simulink library "csu_lnh_ln200_hardware_lib_a"  (R2014b)
settings: Solver=ode45  SolverMode=SingleTasking  StartTime=0.0  StopTime=10.0  RelTol=1e-3
undefined symbols (not defined in the file or in its folder): lnh_accel_range, lnh_accel_SF, lnh_correlation_time, lnh_dt, lnh_gyro_g_sensitive, lnh_gyro_range, lnh_gyro_SF, lnh_gyro_vibe_sensitive
libraries: util_common_lib x7, util_tf_lib x2, util_info_lib x1
settings Model: Creator=hcannon  LastModifiedBy=mstewart

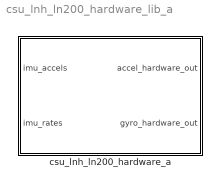
== system csu_lnh_ln200_hardware_lib_a ==
  csu_lnh_ln200_hardware_a : Subsystem

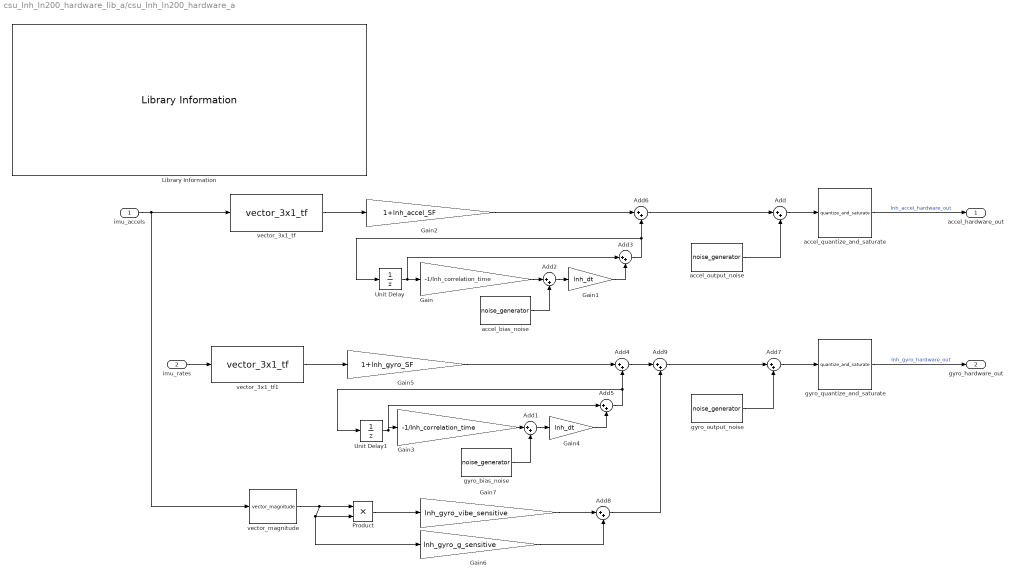
== system csu_lnh_ln200_hardware_lib_a/csu_lnh_ln200_hardware_a ==
  imu_accels : Inport
  imu_rates : Inport  Port=2
  Add{,1..9} (10 alike) : Sum  Inputs=|++
  Gain : Gain  Gain=-1/lnh_correlation_time
  Gain1 : Gain  Gain=lnh_dt
  Gain2 : Gain  Gain=1+lnh_accel_SF
  Gain3 : Gain  Gain=-1/lnh_correlation_time
  Gain4 : Gain  Gain=lnh_dt
  Gain5 : Gain  Gain=1+lnh_gyro_SF
  Gain6 : Gain  Gain=lnh_gyro_g_sensitive
  Gain7 : Gain  Gain=lnh_gyro_vibe_sensitive
  Library Information : util_info_lib/Library Information  owner='NONE'
  Product : Product  RndMeth=Zero
  Unit Delay : UnitDelay  SampleTime=-1
  Unit Delay1 : UnitDelay  SampleTime=-1
  accel_bias_noise : util_common_lib/noise_generator  std_dev=lnh_accel_bias_noise_v  bias=lnh_accel_bias_bias_v  seed=lnh_accel_bias_seed_v  on=lnh_accel_noise_on  sample_time=sim_time_step_size
  accel_output_noise : util_common_lib/noise_generator  std_dev=lnh_accel_noise_v  bias=lnh_accel_bias_v  seed=lnh_accel_seed_v  on=lnh_accel_noise_on  sample_time=sim_time_step_size
  accel_quantize_and_saturate : util_common_lib/quantize_and_saturate  RES=lnh_accel_sensitivity  OPER=truncate  out_min=-lnh_accel_range  out_max=lnh_accel_range
  gyro_bias_noise : util_common_lib/noise_generator  std_dev=lnh_gyro_bias_noise_v  bias=lnh_gyro_bias_bias_v  seed=lnh_gyro_bias_seed_v  on=lnh_gyro_noise_on  sample_time=sim_time_step_size
  gyro_output_noise : util_common_lib/noise_generator  std_dev=lnh_gyro_noise_v  bias=lnh_gyro_bias_v  seed=lnh_gyro_seed_v  on=lnh_gyro_noise_on  sample_time=sim_time_step_size
  gyro_quantize_and_saturate : util_common_lib/quantize_and_saturate  RES=lnh_gyro_sensitivity  OPER=truncate  out_min=-lnh_gyro_range  out_max=lnh_gyro_range
  vector_3x1_tf : util_tf_lib/vector_3x1_tf  num=lnh_accel_response_num  den=lnh_accel_response_den  st=-1
  vector_3x1_tf1 : util_tf_lib/vector_3x1_tf  num=lnh_gyro_response_num  den=lnh_gyro_response_den  st=-1
  vector_magnitude : util_common_lib/vector_magnitude  SystemSampleTime=-1
  accel_hardware_out : Outport
  gyro_hardware_out : Outport  Port=2
  wires:
  Add8/1 -> Add9/2
  Add9/1 -> Add7/1
  Add4/1 -> Add9/1
  Gain6/1 -> Add8/2
  Gain7/1 -> Add8/1
  Product/1 -> Gain7/1
  vector_magnitude/1 -> Gain6/1, Product/2, Product/1
  Add6/1 -> Add/1
  Gain2/1 -> Add6/1
  Gain5/1 -> Add4/1
  Add/1 -> accel_quantize_and_saturate/1
  accel_quantize_and_saturate/1 -> accel_hardware_out/1  "lnh_accel_hardware_out"
  gyro_quantize_and_saturate/1 -> gyro_hardware_out/1  "lnh_gyro_hardware_out"
  imu_accels/1 -> vector_magnitude/1, vector_3x1_tf/1
  imu_rates/1 -> vector_3x1_tf1/1
  accel_output_noise/1 -> Add/2
  Add2/1 -> Gain1/1
  Gain1/1 -> Add3/2
  Unit Delay/1 -> Gain/1, Add3/1
  Add3/1 -> Add6/2, Unit Delay/1
  vector_3x1_tf/1 -> Gain2/1
  Gain/1 -> Add2/1
  accel_bias_noise/1 -> Add2/2
  Add1/1 -> Gain4/1
  Gain4/1 -> Add5/2
  Unit Delay1/1 -> Gain3/1, Add5/1
  Add5/1 -> Add4/2, Unit Delay1/1
  vector_3x1_tf1/1 -> Gain5/1
  Gain3/1 -> Add1/1
  gyro_bias_noise/1 -> Add1/2
  Add7/1 -> gyro_quantize_and_saturate/1
  gyro_output_noise/1 -> Add7/2
